simulink model "On1"  (Simulink 5.0)
settings: Solver=ode45  StartTime=0.0  StopTime=10.0  RelTol=1e-3
settings Model: Creator=scaife  LastModifiedBy=scaife  ExtModeAutoUpdateStatusClock=off

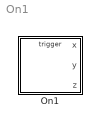
== system On1 ==
  On1 : Stateflow chart

== stateflow chart On1 ==
  state TOP1 [parallel]
    state A
    state B
    A -> B : E/F
    B -> A : E
    (default) -> A
  state TOP2 [parallel]
    state C/
      on F: x++;y++;
      on after (2,E): z++;
    (default) -> C
  data: x output int32; y output int32; z output int32
  events: F local EITHER_EDGE_EVENT; E input EITHER_EDGE_EVENT
